simulink model "bezRegulatora"  (R2019b)
settings: Solver=VariableStepAuto  StartTime=0.0  StopTime=40  RelTol=1e-3
undefined symbols (not defined in the file): k, numerWybranegoWymuszenia, T0, T1, T2, T3, T4, T5
settings Model: Creator=01129847  LastModifiedBy=01129847

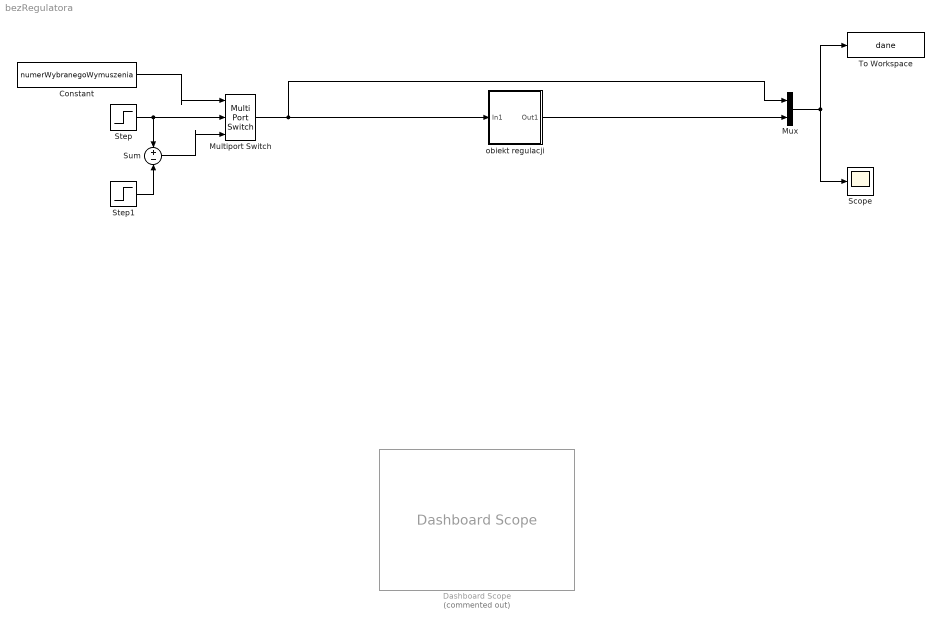
== system bezRegulatora ==
  Constant : Constant  Value=numerWybranegoWymuszenia
  Dashboard Scope : DashboardScope  Commented=on
  Multiport Switch : MultiPortSwitch  Inputs=2
  Mux : Mux  Inputs=2
  Scope : Scope
  Step : Step  Time=10  SampleTime=0
  Step1 : Step  Time=11  SampleTime=0
  Sum : Sum  Inputs=+-
  To Workspace : ToWorkspace  VariableName=dane  SaveFormat=Timeseries  SampleTime=0.1
      settings: Save2DSignal=2-D array (concatenate along first dimension)
  obiekt regulacji : Subsystem
  wires:
  Multiport Switch/1 -> obiekt regulacji/1(In1), Mux/1
  Mux/1 -> To Workspace/1, Scope/1
  Step/1 -> Multiport Switch/2, Sum/1
  Step1/1 -> Sum/2
  Sum/1 -> Multiport Switch/3
  Constant/1 -> Multiport Switch/1
  obiekt regulacji/1(Out1) -> Mux/2

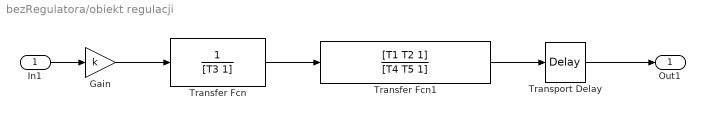
== system bezRegulatora/obiekt regulacji ==
  In1 : Inport
  Gain : Gain  Gain=k
  Transfer Fcn : TransferFcn  Denominator=[T3 1]
  Transfer Fcn1 : TransferFcn  Numerator=[T1 T2 1]  Denominator=[T4 T5 1]
  Transport Delay : TransportDelay  DelayTime=T0
  Out1 : Outport
  wires:
  In1/1 -> Gain/1
  Gain/1 -> Transfer Fcn/1
  Transfer Fcn1/1 -> Transport Delay/1
  Transfer Fcn/1 -> Transfer Fcn1/1
  Transport Delay/1 -> Out1/1
